simulink model "extra_simulink_blocks"  (R2018a)
settings: Solver=VariableStepAuto  StartTime=0.0  StopTime=10.0  RelTol=1e-3
values from neighbouring files (symbols this model uses):
  a1 = 16.235    [QuadrotorConstants.m]    (also in QuadrotorConstants.mat; TuningParameters.mat)
  a2 = 17.912    [QuadrotorConstants.m]    (also in QuadrotorConstants.mat; TuningParameters.mat)
  a3 = 17.914    [QuadrotorConstants.m]    (also in QuadrotorConstants.mat; TuningParameters.mat)
  a4 = 18.161    [QuadrotorConstants.m]    (also in QuadrotorConstants.mat; TuningParameters.mat)
  b1 = -0.5036    [QuadrotorConstants.m]    (also in QuadrotorConstants.mat; TuningParameters.mat)
  b2 = -12.728    [QuadrotorConstants.m]    (also in QuadrotorConstants.mat; TuningParameters.mat)
  b3 = -6.5646    [QuadrotorConstants.m]    (also in QuadrotorConstants.mat; TuningParameters.mat)
  b4 = -7.4637    [QuadrotorConstants.m]    (also in QuadrotorConstants.mat; TuningParameters.mat)
  bb = 2.6846e-07    [QuadrotorConstants.m]    (also in QuadrotorConstants.mat; TuningParameters.mat)
  c = 0.0002    [QuadrotorConstants.m]    (also in QuadrotorConstants.mat; TuningParameters.mat)
  c_mi_x = 1.70    (= 1.7)    [QuadrotorConstants.m]    (also in QuadrotorConstants.mat; TuningParameters.mat)
  c_mi_y = 1.70    (= 1.7)    [QuadrotorConstants.m]    (also in QuadrotorConstants.mat; TuningParameters.mat)
  c_mi_z = 0.40    (= 0.4)    [QuadrotorConstants.m]    (also in QuadrotorConstants.mat; TuningParameters.mat)
  co_x = 1.7    [QuadrotorConstants.m]    (also in QuadrotorConstants.mat; TuningParameters.mat)
  co_y = 1.7    [QuadrotorConstants.m]    (also in QuadrotorConstants.mat; TuningParameters.mat)
  co_z = 3    [QuadrotorConstants.m]    (also in QuadrotorConstants.mat; TuningParameters.mat)
  d = 0.0071    [QuadrotorConstants.m]    (also in QuadrotorConstants.mat; TuningParameters.mat)
  d_omega_R10 = V1_WP    [InitialConditions.m]    (also in TuningParameters.mat = 0.286149195881)
  d_omega_R20 = V2_WP    [InitialConditions.m]    (also in TuningParameters.mat = 0.941828505757)
  d_omega_R30 = V3_WP    [InitialConditions.m]    (also in TuningParameters.mat = 0.597668426656)
  d_omega_R40 = V4_WP    [InitialConditions.m]    (also in TuningParameters.mat = 0.639046979523)
  dd = 2.4481e-03    (= 0.0024481)    [QuadrotorConstants.m]    (also in QuadrotorConstants.mat; TuningParameters.mat)
  dfi_0 = 0    [InitialConditions.m]    (also in TuningParameters.mat)
  disturbancey = 0    [runMain.m]
  disturbancez = 0    [runMain.m]
  dpsi_0 = 0    [InitialConditions.m]    (also in TuningParameters.mat)
  dtheta_0 = 0    [InitialConditions.m]    (also in TuningParameters.mat)
  dx_0 = 0    [InitialConditions.m]    (also in TuningParameters.mat)
  dy_0 = 0    [InitialConditions.m]    (also in TuningParameters.mat)
  dz_0 = 5    [InitialConditions.m]    (also in TuningParameters.mat)
  f = 5e-6    (= 5e-06)    [QuadrotorConstants.m]    (also in QuadrotorConstants.mat; TuningParameters.mat; animateQuadrotor.m = getframe; animateQuadrotorConstant.m = getframe)
  fi_0 = pi    (= 3.14159265359)    [InitialConditions.m]    (also in TuningParameters.mat)
  g = 0.0008    [QuadrotorConstants.m]    (also in QuadrotorConstants.mat; TuningParameters.mat)
  ga = 9.807    [QuadrotorConstants.m]    (also in QuadrotorConstants.mat; TuningParameters.mat)
  h = -0.0282    [QuadrotorConstants.m]    (also in QuadrotorConstants.mat; TuningParameters.mat)
  Ixx = 2.1385*1    (= 2.1385)    [QuadrotorConstants.m]    (also in QuadrotorConstants.mat; TuningParameters.mat)
  Iyy = Ixx    (= 2.1385)    [QuadrotorConstants.m]    (also in QuadrotorConstants.mat; TuningParameters.mat)
  Izz = 3.7479*1    (= 3.7479)    [QuadrotorConstants.m]    (also in QuadrotorConstants.mat; TuningParameters.mat)
  Jr = 4.86851*0.1    (= 0.486851)    [QuadrotorConstants.m]    (also in QuadrotorConstants.mat; TuningParameters.mat)
  L = 0.422    [QuadrotorConstants.m]    (also in QuadrotorConstants.mat; TuningParameters.mat)
  m = 2.1    [QuadrotorConstants.m]    (also in QuadrotorConstants.mat; TuningParameters.mat)
  psi_0 = 0    [InitialConditions.m]    (also in TuningParameters.mat)
  Tau = 0.1    [QuadrotorConstants.m]    (also in QuadrotorConstants.mat; TuningParameters.mat)
  theta_0 = 0    [InitialConditions.m]    (also in TuningParameters.mat)
  x_0 = 0    [InitialConditions.m]    (also in TuningParameters.mat)
  XDes = [t,xdes,dxdes,ydes,dydes,zdes,dzdes,phides,dphides,thetades,dthetades,psides,dpsides]    [runMain.m]
  y_0 = 0    [InitialConditions.m]    (also in TuningParameters.mat)
  z_0 = 10    [InitialConditions.m]    (also in TuningParameters.mat)
undefined symbols (not defined in the file or in its folder): maxdz, sigbuilder_block, X, Y, Z
libraries: sm_lib x34, nesl_utility x21
(part 2 of 2)

== system extra_simulink_blocks/Dynamics1/Body dynamics ==
  U1 : Inport
  U2 : Inport  Port=2
  U3 : Inport  Port=3
  U4 : Inport  Port=4
  Omega : Inport  Port=5
  Mux : Mux  Inputs=6
  Pitch Stability : Subsystem
  Position Stability : Subsystem
  Roll Stability : Subsystem
  Yaw Stability : Subsystem
  Position : Outport
  Orientation : Outport  Port=2
  wires:
  U4/1 -> Yaw Stability/1(U4)
  U3/1 -> Pitch Stability/3(U3)
  U1/1 -> Position Stability/1(U1)
  U2/1 -> Roll Stability/2(U2)
  Omega/1 -> Pitch Stability/2(SumYRtrSpd), Roll Stability/1(SumXRtrSpd)
  Roll Stability/1(Phi) -> Mux/1, Position Stability/2(fi)
  Pitch Stability/1(Theta) -> Position Stability/3(theta), Mux/3
  Yaw Stability/1(Psi) -> Position Stability/4(psi), Mux/5
  Roll Stability/2(dPhi) -> Mux/2, Yaw Stability/2(dPhi), Pitch Stability/1(dPhi)
  Yaw Stability/2(dPsi) -> Roll Stability/4(dPsi), Pitch Stability/4(dPsi), Mux/6
  Pitch Stability/2(dTheta) -> Yaw Stability/3(dTheta), Roll Stability/3(dTheta), Mux/4
  Position Stability/1(Position) -> Position/1
  Mux/1 -> Orientation/1

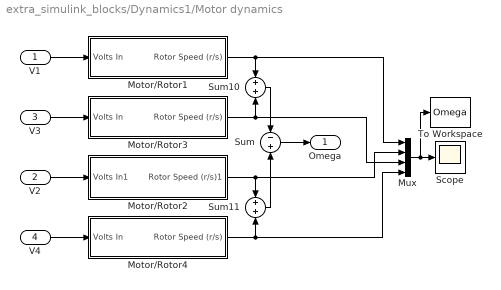
== system extra_simulink_blocks/Dynamics1/Motor dynamics ==
  V1 : Inport
  V2 : Inport  Port=2
  V3 : Inport  Port=3
  V4 : Inport  Port=4
  Motor/Rotor1 : Subsystem
  Motor/Rotor2 : Subsystem
  Motor/Rotor3 : Subsystem
  Motor/Rotor4 : Subsystem
  Mux : Mux
  Scope : Scope
  Sum : Sum  Inputs=-+
  Sum10 : Sum  Inputs=+|+
  Sum11 : Sum  Inputs=+|+
  To Workspace : ToWorkspace  VariableName=Omega  SaveFormat=Timeseries  SampleTime=-1
  Omega : Outport
  wires:
  Sum11/1 -> Sum/2
  Sum10/1 -> Sum/1
  Motor/Rotor4/1(Rotor Speed (r/s)) -> Mux/4, Sum11/2
  Motor/Rotor3/1(Rotor Speed (r/s)) -> Mux/3, Sum10/2
  Motor/Rotor2/1(Rotor Speed (r/s)1) -> Mux/2, Sum11/1
  Motor/Rotor1/1(Rotor Speed (r/s)) -> Mux/1, Sum10/1
  Sum/1 -> Omega/1
  V1/1 -> Motor/Rotor1/1(Volts In)
  V4/1 -> Motor/Rotor4/1(Volts In)
  V3/1 -> Motor/Rotor3/1(Volts In)
  V2/1 -> Motor/Rotor2/1(Volts In1)
  Mux/1 -> To Workspace/1, Scope/1

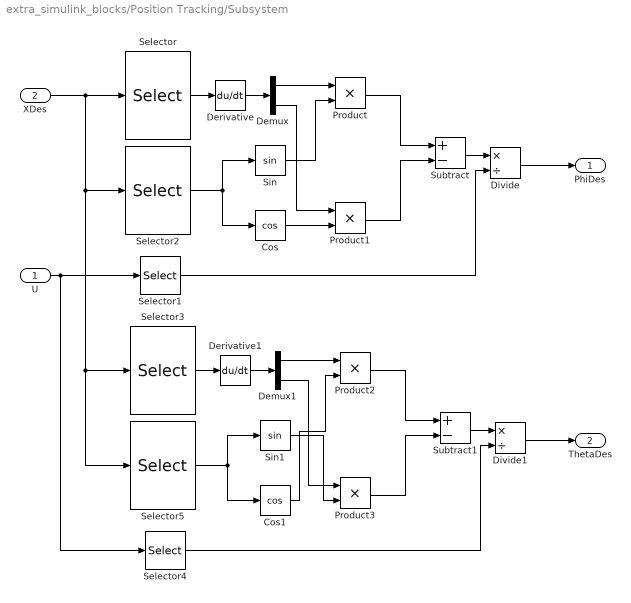
== system extra_simulink_blocks/Position Tracking/Subsystem ==
  U : Inport
  XDes : Inport  Port=2
  Cos : Trigonometry  Operator=cos
  Cos1 : Trigonometry  Operator=cos
  Demux : Demux  Outputs=2
  Demux1 : Demux  Outputs=2
  Derivative : Derivative
  Derivative1 : Derivative
  Divide : Product  Inputs=*/
  Divide1 : Product  Inputs=*/
  Product{,1..3} (4 alike) : Product
  Selector : Selector  InputPortWidth=12  IndexOptions=Index vector (dialog)  Indices=[2 4]  OutputSizes=1
  Selector1 : Selector  InputPortWidth=4  IndexOptions=Index vector (dialog)  Indices=[1]  OutputSizes=1
  Selector2 : Selector  InputPortWidth=12  IndexOptions=Index vector (dialog)  Indices=[11]  OutputSizes=1
  Selector3 : Selector  InputPortWidth=12  IndexOptions=Index vector (dialog)  Indices=[2 4]  OutputSizes=1
  Selector4 : Selector  InputPortWidth=4  IndexOptions=Index vector (dialog)  Indices=[1]  OutputSizes=1
  Selector5 : Selector  InputPortWidth=12  IndexOptions=Index vector (dialog)  Indices=[11]  OutputSizes=1
  Sin : Trigonometry
  Sin1 : Trigonometry
  Subtract : Sum  Inputs=+-
  Subtract1 : Sum  Inputs=+-
  PhiDes : Outport
  ThetaDes : Outport  Port=2
  wires:
  Derivative/1 -> Demux/1
  Selector/1 -> Derivative/1
  Demux/1 -> Product/1
  XDes/1 -> Selector5/1, Selector3/1, Selector2/1, Selector/1
  Cos/1 -> Product1/2
  Product/1 -> Subtract/1
  Product1/1 -> Subtract/2
  Subtract/1 -> Divide/1
  Divide/1 -> PhiDes/1
  Selector1/1 -> Divide/2
  Selector2/1 -> Cos/1, Sin/1
  Demux/2 -> Product1/1
  Sin/1 -> Product/2
  Selector3/1 -> Derivative1/1
  Product3/1 -> Subtract1/2
  Selector4/1 -> Divide1/2
  Product2/1 -> Subtract1/1
  U/1 -> Selector4/1, Selector1/1
  Divide1/1 -> ThetaDes/1
  Derivative1/1 -> Demux1/1
  Selector5/1 -> Cos1/1, Sin1/1
  Subtract1/1 -> Divide1/1
  Sin1/1 -> Product3/2
  Cos1/1 -> Product2/2
  Demux1/1 -> Product2/1
  Demux1/2 -> Product3/1

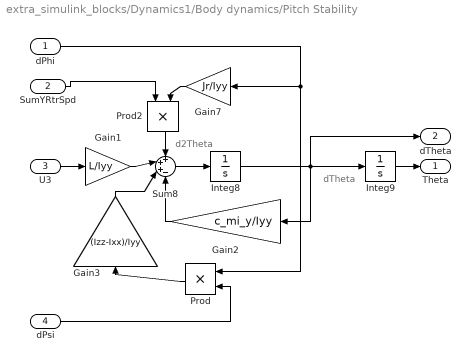
== system extra_simulink_blocks/Dynamics1/Body dynamics/Pitch Stability ==
  note: d2Theta
  note: dTheta
  dPhi : Inport
  SumYRtrSpd : Inport  Port=2
  U3 : Inport  Port=3
  dPsi : Inport  Port=4
  Gain1 : Gain  Gain=L/Iyy
  Gain2 : Gain  Gain=c_mi_y/Iyy
  Gain3 : Gain  Gain=(Izz-Ixx)/Iyy
  Gain7 : Gain  Gain=Jr/Iyy
  Integ8 : Integrator  InitialCondition=dtheta_0
  Integ9 : Integrator  InitialCondition=theta_0  UpperSaturationLimit=pi/2  LowerSaturationLimit=-pi/2
  Prod : Product  RndMeth=Zero
  Prod2 : Product  RndMeth=Zero
  Sum8 : Sum  Inputs=+++-
  Theta : Outport
  dTheta : Outport  Port=2
  wires:
  Gain2/1 -> Sum8/4
  dPhi/1 -> Prod/1, Gain7/1
  Integ9/1 -> Theta/1
  U3/1 -> Gain1/1
  SumYRtrSpd/1 -> Prod2/1
  dPsi/1 -> Prod/2
  Integ8/1 -> dTheta/1, Integ9/1, Gain2/1
  Sum8/1 -> Integ8/1
  Gain1/1 -> Sum8/2
  Gain7/1 -> Prod2/2
  Gain3/1 -> Sum8/3
  Prod/1 -> Gain3/1
  Prod2/1 -> Sum8/1

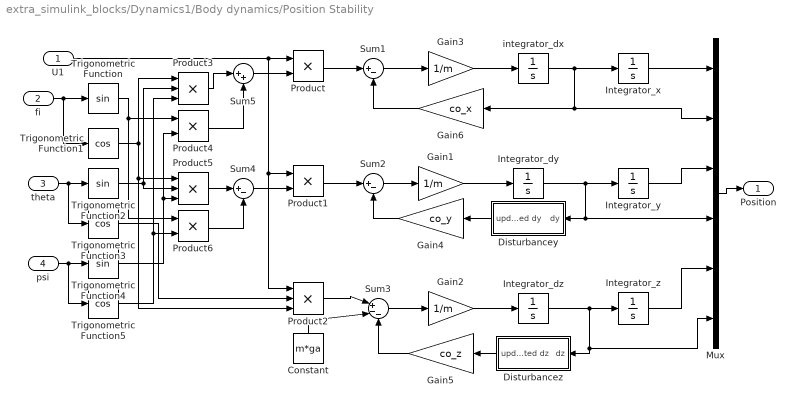
== system extra_simulink_blocks/Dynamics1/Body dynamics/Position Stability ==
  U1 : Inport
  fi : Inport  Port=2
  theta : Inport  Port=3
  psi : Inport  Port=4
  Constant : Constant  Value=m*ga
  Disturbancey : Subsystem
  Disturbancez : Subsystem
  Gain1 : Gain  Gain=1/m
  Gain2 : Gain  Gain=1/m
  Gain3 : Gain  Gain=1/m
  Gain4 : Gain  Gain=co_y
  Gain5 : Gain  Gain=co_z
  Gain6 : Gain  Gain=co_x
  Integrator_dy : Integrator  InitialCondition=dy_0  LimitOutput=on  UpperSaturationLimit=1000  LowerSaturationLimit=-1000
  Integrator_dz : Integrator  InitialCondition=dz_0  LimitOutput=on  UpperSaturationLimit=1000  LowerSaturationLimit=-1000
  Integrator_x : Integrator  InitialCondition=x_0
  Integrator_y : Integrator  InitialCondition=y_0
  Integrator_z : Integrator  InitialCondition=z_0
  Mux : Mux  Inputs=6
  Product{,1,4,6} (4 alike) : Product  RndMeth=Zero
  Product2 : Product  Inputs=3  RndMeth=Zero
  Product3 : Product  Inputs=3  RndMeth=Zero
  Product5 : Product  Inputs=3  RndMeth=Zero
  Sum1 : Sum  Inputs=|+-
  Sum2 : Sum  Inputs=|+-
  Sum3 : Sum  Inputs=|+--
  Sum4 : Sum  Inputs=|+-
  Sum5 : Sum  Inputs=|++
  Trigonometric Function : Trigonometry
  Trigonometric Function1 : Trigonometry  Operator=cos
  Trigonometric Function2 : Trigonometry
  Trigonometric Function3 : Trigonometry  Operator=cos
  Trigonometric Function4 : Trigonometry
  Trigonometric Function5 : Trigonometry  Operator=cos
  integrator_dx : Integrator  InitialCondition=dx_0  LimitOutput=on  UpperSaturationLimit=1000  LowerSaturationLimit=-1000
  Position : Outport
  wires:
  Gain5/1 -> Sum3/3
  Constant/1 -> Sum3/2
  Gain4/1 -> Sum2/2
  Sum3/1 -> Gain2/1
  Gain6/1 -> Sum1/2
  Product2/1 -> Sum3/1
  Sum2/1 -> Gain1/1
  Product1/1 -> Sum2/1
  Gain2/1 -> Integrator_dz/1
  Sum1/1 -> Gain3/1
  Product/1 -> Sum1/1
  U1/1 -> Product/1, Product1/1, Product2/1
  Integrator_x/1 -> Mux/1
  integrator_dx/1 -> Integrator_x/1, Mux/2, Gain6/1
  Integrator_dy/1 -> Integrator_y/1, Disturbancey/1(dy), Mux/4
  Integrator_dz/1 -> Integrator_z/1, Disturbancez/1(dz), Mux/6
  Gain1/1 -> Integrator_dy/1
  Gain3/1 -> integrator_dx/1
  Sum4/1 -> Product1/2
  Sum5/1 -> Product/2
  Product3/1 -> Sum5/1
  Product4/1 -> Sum5/2
  Product5/1 -> Sum4/1
  Product6/1 -> Sum4/2
  psi/1 -> Trigonometric Function4/1, Trigonometric Function5/1
  theta/1 -> Trigonometric Function2/1, Trigonometric Function3/1
  fi/1 -> Trigonometric Function/1, Trigonometric Function1/1
  Trigonometric Function/1 -> Product4/1, Product6/1
  Trigonometric Function1/1 -> Product3/1, Product5/1, Product2/3
  Trigonometric Function2/1 -> Product3/2, Product5/2
  Trigonometric Function5/1 -> Product3/3, Product6/2
  Trigonometric Function4/1 -> Product4/2, Product5/3
  Trigonometric Function3/1 -> Product2/2
  Integrator_y/1 -> Mux/3
  Integrator_z/1 -> Mux/5
  Mux/1 -> Position/1
  Disturbancez/1(updated dz) -> Gain5/1
  Disturbancey/1(updated dy) -> Gain4/1

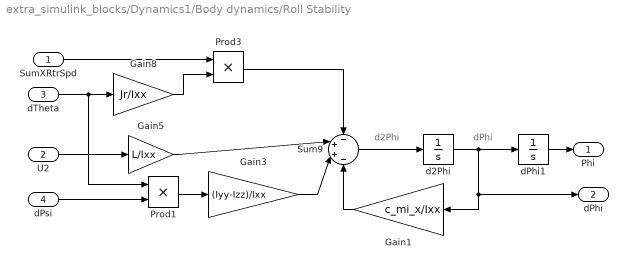
== system extra_simulink_blocks/Dynamics1/Body dynamics/Roll Stability ==
  note: d2Phi
  note: dPhi
  SumXRtrSpd : Inport
  U2 : Inport  Port=2
  dTheta : Inport  Port=3
  dPsi : Inport  Port=4
  Gain1 : Gain  Gain=c_mi_x/Ixx
  Gain3 : Gain  Gain=(Iyy-Izz)/Ixx
  Gain5 : Gain  Gain=L/Ixx
  Gain8 : Gain  Gain=Jr/Ixx
  Prod1 : Product  RndMeth=Zero
  Prod3 : Product  RndMeth=Zero
  Sum9 : Sum  Inputs=-++-
  d2Phi : Integrator  InitialCondition=dfi_0
  dPhi1 : Integrator  InitialCondition=fi_0  UpperSaturationLimit=pi/2  LowerSaturationLimit=-pi/2
  Phi : Outport
  dPhi : Outport  Port=2
  wires:
  dPsi/1 -> Prod1/2
  dTheta/1 -> Prod1/1, Gain8/1
  Prod3/1 -> Sum9/1
  SumXRtrSpd/1 -> Prod3/1
  Gain8/1 -> Prod3/2
  dPhi1/1 -> Phi/1
  U2/1 -> Gain5/1
  d2Phi/1 -> Gain1/1, dPhi/1, dPhi1/1
  Sum9/1 -> d2Phi/1
  Gain5/1 -> Sum9/2
  Gain1/1 -> Sum9/4
  Gain3/1 -> Sum9/3
  Prod1/1 -> Gain3/1

== system extra_simulink_blocks/Dynamics1/Body dynamics/Yaw Stability ==
  note: dPsi
  note: d2Psi
  U4 : Inport
  dPhi : Inport  Port=2
  dTheta : Inport  Port=3
  Gain : Gain  Gain=1/Izz
  Gain1 : Gain  Gain=c_mi_z
  Gain2 : Gain  Gain=Ixx-Iyy
  Integ10 : Integrator  InitialCondition=dpsi_0
  Integ11 : Integrator  InitialCondition=psi_0
  Product : Product  RndMeth=Zero
  Sum : Sum  Inputs=|++-
  Psi : Outport
  dPsi : Outport  Port=2
  wires:
  Sum/1 -> Gain/1
  U4/1 -> Sum/1
  Integ11/1 -> Psi/1
  Gain/1 -> Integ10/1
  Integ10/1 -> Gain1/1, dPsi/1, Integ11/1
  Gain1/1 -> Sum/3
  Gain2/1 -> Sum/2
  dPhi/1 -> Product/1
  dTheta/1 -> Product/2
  Product/1 -> Gain2/1

== system extra_simulink_blocks/Dynamics1/Motor dynamics/Motor//Rotor1 ==
  note: Omega1
      | (r/s)
  Volts In : Inport
  DragFcn1 : Fcn  Commented=on  Expr=dd*u^2
  Gain : Gain  Gain=1/Tau
  Integrator : Integrator  InitialCondition=d_omega_R10
  RtrSpdFcn1 : Fcn  Expr=a1*u+b1
  Saturation3 : Saturate  Commented=on  UpperLimit=1000  LowerLimit=-1000
  Saturation4 : Saturate  UpperLimit=250  LowerLimit=0
  Saturation8 : Saturate  Commented=on  UpperLimit=1000  LowerLimit=-1000
  Sum : Sum  Inputs=|+-
  ThrustFcn1 : Fcn  Commented=on  Expr=bb*u^2
  r/s 2 rpm : Gain  Commented=on  Gain=60/2/pi
  r/s 2 rpm1 : Gain  Commented=on  Gain=60/2/pi
  Rotor Speed (r/s) : Outport
  wires:
  Volts In/1 -> Sum/1
  Sum/1 -> Gain/1
  Integrator/1 -> RtrSpdFcn1/1, Sum/2
  Gain/1 -> Integrator/1
  DragFcn1/1 -> Saturation8/1
  RtrSpdFcn1/1 -> Saturation4/1
  ThrustFcn1/1 -> Saturation3/1
  Saturation4/1 -> Rotor Speed (r/s)/1, r/s 2 rpm1/1, r/s 2 rpm/1
  r/s 2 rpm/1 -> ThrustFcn1/1
  r/s 2 rpm1/1 -> DragFcn1/1

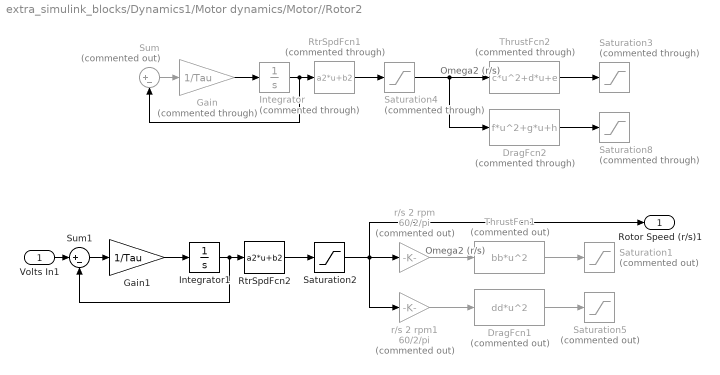
== system extra_simulink_blocks/Dynamics1/Motor dynamics/Motor//Rotor2 ==
  note: Omega2
      | (r/s)
  note: Omega2
      | (r/s)
  Volts In1 : Inport
  DragFcn1 : Fcn  Commented=on  Expr=dd*u^2
  DragFcn2 : Fcn  Commented=through  Expr=f*u^2+g*u+h
  Gain : Gain  Commented=through  Gain=1/Tau
  Gain1 : Gain  Gain=1/Tau
  Integrator : Integrator  Commented=through  InitialCondition=d_omega_R20
  Integrator1 : Integrator  InitialCondition=d_omega_R20
  RtrSpdFcn1 : Fcn  Commented=through  Expr=a2*u+b2
  RtrSpdFcn2 : Fcn  Expr=a2*u+b2
  Saturation1 : Saturate  Commented=on  UpperLimit=1000  LowerLimit=-1000
  Saturation2 : Saturate  UpperLimit=250  LowerLimit=0
  Saturation3 : Saturate  Commented=through  UpperLimit=1000  LowerLimit=-1000
  Saturation4 : Saturate  Commented=through  UpperLimit=1000  LowerLimit=-1000
  Saturation5 : Saturate  Commented=on  UpperLimit=1000  LowerLimit=-1000
  Saturation8 : Saturate  Commented=through  UpperLimit=1000  LowerLimit=-1000
  Sum : Sum  Commented=on  Inputs=|+-
  Sum1 : Sum  Inputs=|+-
  ThrustFcn1 : Fcn  Commented=on  Expr=bb*u^2
  ThrustFcn2 : Fcn  Commented=through  Expr=c*u^2+d*u+e
  r/s 2 rpm : Gain  Commented=on  Gain=60/2/pi
  r/s 2 rpm1 : Gain  Commented=on  Gain=60/2/pi
  Rotor Speed (r/s)1 : Outport
  wires:
  Sum/1 -> Gain/1
  Integrator/1 -> RtrSpdFcn1/1, Sum/2
  Gain/1 -> Integrator/1
  RtrSpdFcn1/1 -> Saturation4/1
  ThrustFcn2/1 -> Saturation3/1
  Saturation4/1 -> DragFcn2/1, ThrustFcn2/1
  DragFcn2/1 -> Saturation8/1
  DragFcn1/1 -> Saturation5/1
  Integrator1/1 -> RtrSpdFcn2/1, Sum1/2
  Gain1/1 -> Integrator1/1
  RtrSpdFcn2/1 -> Saturation2/1
  ThrustFcn1/1 -> Saturation1/1
  Volts In1/1 -> Sum1/1
  Sum1/1 -> Gain1/1
  Saturation2/1 -> Rotor Speed (r/s)1/1, r/s 2 rpm1/1, r/s 2 rpm/1
  r/s 2 rpm1/1 -> DragFcn1/1
  r/s 2 rpm/1 -> ThrustFcn1/1

== system extra_simulink_blocks/Dynamics1/Motor dynamics/Motor//Rotor3 ==
  note: Omega3
      | (r/s)
  Volts In : Inport
  DragFcn3 : Fcn  Commented=on  Expr=dd*u^2
  Gain : Gain  Gain=1/Tau
  Integrator : Integrator  InitialCondition=d_omega_R30
  RtrSpdFcn3 : Fcn  Expr=a3*u+b3
  Saturation3 : Saturate  Commented=on  UpperLimit=1000  LowerLimit=-1000
  Saturation4 : Saturate  UpperLimit=250  LowerLimit=0
  Saturation8 : Saturate  Commented=on  UpperLimit=1000  LowerLimit=-1000
  Sum : Sum  Inputs=|+-
  ThrustFcn3 : Fcn  Commented=on  Expr=bb*u^2
  r/s 2 rpm : Gain  Commented=on  Gain=60/2/pi
  r/s 2 rpm1 : Gain  Commented=on  Gain=60/2/pi
  Rotor Speed (r/s) : Outport
  wires:
  Volts In/1 -> Sum/1
  Sum/1 -> Gain/1
  Integrator/1 -> RtrSpdFcn3/1, Sum/2
  Gain/1 -> Integrator/1
  RtrSpdFcn3/1 -> Saturation4/1
  ThrustFcn3/1 -> Saturation3/1
  DragFcn3/1 -> Saturation8/1
  Saturation4/1 -> Rotor Speed (r/s)/1, r/s 2 rpm1/1, r/s 2 rpm/1
  r/s 2 rpm/1 -> ThrustFcn3/1
  r/s 2 rpm1/1 -> DragFcn3/1

== system extra_simulink_blocks/Dynamics1/Motor dynamics/Motor//Rotor4 ==
  note: Omega1
      | (r/s)
  Volts In : Inport
  DragFcn4 : Fcn  Commented=on  Expr=dd*u^2
  Gain : Gain  Gain=1/Tau
  Integrator : Integrator  InitialCondition=d_omega_R40
  RtrSpdFcn4 : Fcn  Expr=a4*u+b4
  Saturation3 : Saturate  Commented=on  UpperLimit=1000  LowerLimit=-1000
  Saturation4 : Saturate  UpperLimit=250  LowerLimit=0
  Saturation8 : Saturate  Commented=on  UpperLimit=1000  LowerLimit=-1000
  Sum : Sum  Inputs=|+-
  ThrustFcn4 : Fcn  Commented=on  Expr=bb*u^2
  r/s 2 rpm : Gain  Commented=on  Gain=60/2/pi
  r/s 2 rpm1 : Gain  Commented=on  Gain=60/2/pi
  Rotor Speed (r/s) : Outport
  wires:
  Volts In/1 -> Sum/1
  Sum/1 -> Gain/1
  Integrator/1 -> RtrSpdFcn4/1, Sum/2
  Gain/1 -> Integrator/1
  RtrSpdFcn4/1 -> Saturation4/1
  ThrustFcn4/1 -> Saturation3/1
  DragFcn4/1 -> Saturation8/1
  Saturation4/1 -> Rotor Speed (r/s)/1, r/s 2 rpm1/1, r/s 2 rpm/1
  r/s 2 rpm/1 -> ThrustFcn4/1
  r/s 2 rpm1/1 -> DragFcn4/1

== system extra_simulink_blocks/Dynamics1/Body dynamics/Position Stability/Disturbancey ==
  dy : Inport
  Constant1 : Constant  Value=disturbancey
  If : If  IfExpression=u1 == 1
  If Action Subsystem : Subsystem  TreatAsAtomicUnit=on
  If Action Subsystem1 : Subsystem  TreatAsAtomicUnit=on
  Merge : Merge
  updated dy : Outport
  wires:
  If Action Subsystem/1(updated dy) -> Merge/1
  If Action Subsystem1/1(updated dz) -> Merge/2
  Merge/1 -> updated dy/1
  If/2 -> If Action Subsystem1/Action
  Constant1/1 -> If/1
  If/1 -> If Action Subsystem/Action
  dy/1 -> If Action Subsystem/1(dy), If Action Subsystem1/1(dz)

== system extra_simulink_blocks/Dynamics1/Body dynamics/Position Stability/Disturbancez ==
  dz : Inport
  Constant1 : Constant  Value=disturbancez
  If : If  IfExpression=u1 == 1
  If Action Subsystem : Subsystem  TreatAsAtomicUnit=on
  If Action Subsystem1 : Subsystem  TreatAsAtomicUnit=on
  Merge : Merge
  updated dz : Outport
  wires:
  If Action Subsystem/1(updated dz) -> Merge/1
  If Action Subsystem1/1(updated dz) -> Merge/2
  Merge/1 -> updated dz/1
  If/2 -> If Action Subsystem1/Action
  Constant1/1 -> If/1
  If/1 -> If Action Subsystem/Action
  dz/1 -> If Action Subsystem/1(dz), If Action Subsystem1/1(dz)

== system extra_simulink_blocks/Dynamics1/Body dynamics/Position Stability/Disturbancey/If Action Subsystem ==
  dy : Inport
  Action Port : ActionPort
  add disturbance : Subsystem
  updated dy : Outport
  wires:
  dy/1 -> add disturbance/1(dy)
  add disturbance/1(updated dy) -> updated dy/1

== system extra_simulink_blocks/Dynamics1/Body dynamics/Position Stability/Disturbancey/If Action Subsystem1 ==
  dz : Inport
  Action Port : ActionPort
  updated dz : Outport
  wires:
  dz/1 -> updated dz/1

== system extra_simulink_blocks/Dynamics1/Body dynamics/Position Stability/Disturbancez/If Action Subsystem ==
  dz : Inport
  Action Port : ActionPort
  add disturbance : Subsystem
  updated dz : Outport
  wires:
  dz/1 -> add disturbance/1(dz)
  add disturbance/1(updated dz) -> updated dz/1

== system extra_simulink_blocks/Dynamics1/Body dynamics/Position Stability/Disturbancez/If Action Subsystem1 ==
  dz : Inport
  Action Port : ActionPort
  updated dz : Outport
  wires:
  dz/1 -> updated dz/1

== system extra_simulink_blocks/Dynamics1/Body dynamics/Position Stability/Disturbancey/If Action Subsystem/add disturbance ==
  dy : Inport
  Subtract : Sum  Inputs=-+
  "vwind " : Subsystem
  updated dy : Outport
  wires:
  dy/1 -> Subtract/2
  "vwind "/1(vwind) -> Subtract/1
  Subtract/1 -> updated dy/1

== system extra_simulink_blocks/Dynamics1/Body dynamics/Position Stability/Disturbancez/If Action Subsystem/add disturbance ==
  dz : Inport
  Subtract : Sum  Inputs=-+
  "vwind " : Subsystem
  updated dz : Outport
  wires:
  dz/1 -> Subtract/2
  "vwind "/1(vwind) -> Subtract/1
  Subtract/1 -> updated dz/1

== system extra_simulink_blocks/Dynamics1/Body dynamics/Position Stability/Disturbancey/If Action Subsystem/add disturbance/vwind  ==
  Signal Builder : Subsystem  Tag=STV Subsys  LoadFcn=sigbuilder_block('load');  StartFcn=sigbuilder_block('start');  StopFcn=sigbuilder_block('stop');  ClipboardFcn=sigbuilder_block('clipboard');  mask(Sigbuilder block){tuvar=[0:10]}
      mask help: Simulink:masks:SigbuilderBlock_MD
      mask init:
      | if ~strcmp(get_param(bdroot(gcbh),'SimulationStatus'),'stopped') tuvar = sigbuilder_block('maskInit'); end
      settings: CopyFcn=sigbuilder_block('copy');  DeleteFcn=sigbuilder_block('delete');  ModelCloseFcn=sigbuilder_block('modelClose');  PreSaveFcn=sigbuilder_block('preSave');  PauseFcn=sigbuilder_block('pause');  ContinueFcn=sigbuilder_block('continue');  NameChangeFcn=sigbuilder_block('namechange');  OpenFcn=sigbuilder_block('open',[394.2 102 550.8 400.2 ]);  CloseFcn=sigbuilder_block('close');
      mask Display: plot(0, 0, 100, 100,[2, 2, 32, 32, 2], [68, 8, 8, 68, 68],[32, 2], [38, 38], [32, 19, 2],[53, 60, 44], [32, 17, 17, 2],[16, 16, 31, 31]);txt = getActiveGroup(gcbh);text(2, 100, txt,'verticalAlignment', 'top');
  vwind : Outport
  wires:
  Signal Builder/1(Signal 1) -> vwind/1

== system extra_simulink_blocks/Dynamics1/Body dynamics/Position Stability/Disturbancez/If Action Subsystem/add disturbance/vwind  ==
  note: step down
  note: step up
  Add : Sum  Commented=on
  Signal Builder : Subsystem  Tag=STV Subsys  LoadFcn=sigbuilder_block('load');  StartFcn=sigbuilder_block('start');  StopFcn=sigbuilder_block('stop');  ClipboardFcn=sigbuilder_block('clipboard');  mask(Sigbuilder block){tuvar=[0:10]}
      mask help: Simulink:masks:SigbuilderBlock_MD
      mask init:
      | if ~strcmp(get_param(bdroot(gcbh),'SimulationStatus'),'stopped') tuvar = sigbuilder_block('maskInit'); end
      settings: CopyFcn=sigbuilder_block('copy');  DeleteFcn=sigbuilder_block('delete');  ModelCloseFcn=sigbuilder_block('modelClose');  PreSaveFcn=sigbuilder_block('preSave');  PauseFcn=sigbuilder_block('pause');  ContinueFcn=sigbuilder_block('continue');  NameChangeFcn=sigbuilder_block('namechange');  OpenFcn=sigbuilder_block('open',[437.6 199.2 550.4 400 ]);  CloseFcn=sigbuilder_block('close');
      mask Display: plot(0, 0, 100, 100,[2, 2, 32, 32, 2], [68, 8, 8, 68, 68],[32, 2], [38, 38], [32, 19, 2],[53, 60, 44], [32, 17, 17, 2],[16, 16, 31, 31]);txt = getActiveGroup(gcbh);text(2, 100, txt,'verticalAlignment', 'top');
  Step : Step  Commented=on  Time=2  After=maxdz  SampleTime=0
  Step1 : Step  Commented=on  Time=2.25  After=-maxdz  SampleTime=0
  vwind : Outport
  wires:
  Signal Builder/1(Signal 1) -> vwind/1
  Step/1 -> Add/1
  Step1/1 -> Add/2

== system extra_simulink_blocks/Dynamics1/Body dynamics/Position Stability/Disturbancey/If Action Subsystem/add disturbance/vwind /Signal Builder ==
  Demux : Demux  Tag=STV Demux  Outputs=1
  FromWs : FromWorkspace  Tag=STV FromWs  VariableName=tuvar  SampleTime=0
      SigBuilderData=|
      | common.afterFinalStr = 'Extrapolate'
      | common.sampleTime = 0
      | dataSet.timeRange = [0 10]
      | dataSet.name = 'Group 1'
      | sbobj.Groups.Name = 'Group 1'
      | sbobj.Groups.Signals.Name = 'Signal 1'
      | sbobj.Groups.Signals.XData = [0 2 2 2.001 10]
      | sbobj.Groups.Signals.YData = [0 0 10000 0 0]
  Signal 1 : Outport  Tag=STV Outport
  wires:
  Demux/1 -> Signal 1/1
  FromWs/1 -> Demux/1

== system extra_simulink_blocks/Dynamics1/Body dynamics/Position Stability/Disturbancez/If Action Subsystem/add disturbance/vwind /Signal Builder ==
  Demux : Demux  Tag=STV Demux  Outputs=1
  FromWs : FromWorkspace  Tag=STV FromWs  VariableName=tuvar  SampleTime=0
      SigBuilderData=|
      | common.afterFinalStr = 'Extrapolate'
      | common.sampleTime = 0
      | dataSet.timeRange = [0 10]
      | dataSet.name = 'Group 1'
      | sbobj.Groups.Name = 'Group 1'
      | sbobj.Groups.Signals.Name = 'Signal 1'
      | sbobj.Groups.Signals.XData = [0 2 2 2.001 10]
      | sbobj.Groups.Signals.YData = [0 0 10000 0 0]
  Signal 1 : Outport  Tag=STV Outport
  wires:
  Demux/1 -> Signal 1/1
  FromWs/1 -> Demux/1

== matlab function extra_simulink_blocks/Controller1/calculateU ==
  data: x input; u output; xd input; om input; s output
function [u,s] = fcn(x,xd,om)

% load parameters
p = load('QuadrotorConstants'); % Load quadrotor constants
t = load('TuningParameters');   % Load tuning parameters

% initialize memory for u and s
u = zeros(4,1);
s = zeros(4,1);

% store state into smaller variables
X   = [ x(5)  x(7)  x(9)   x(11)].';
dX  = [ x(6)  x(8)  x(10)  x(12)].';
Xd  = [xd(5) xd(7) xd(9)  xd(11)].';
% dXd = [xd(6) xd(8) xd(10) xd(12)].';

% find desired derivatives
dXd = (Xd-X)./t.tau;
% dXd(2:4) = 1e-6*dXd(2:4);
ddXd = (dXd-dX)./t.tau;

% sliding surfaces
s = t.lambda.*(Xd-X) + (dXd-dX);

% find the sign / sigmoid of sliding surfaces
sigma = tanh(s);

% find the derivatives of sliding surfaces
ds = - t.K.*sigma - t.eta.*s;

% find the EOMs from the sliding surfaces
% ddx = zeros(4,1);
ddX = - ds + t.lambda.*(dXd - dX) + ddXd;

% find which state should be controlled
% s(~cont) = 0;

% find the inputs
% if s(1) ~= 0
%     u(1) = ( p.m/cos(X(2))/cos(X(3)) ) * ...
%         ( p.ga + ddX(1));
% end
% if s(2) ~= 0
%     u(2) = (p.Ixx/p.L) * ( - ((p.Iyy-p.Izz)/(p.Ixx))*dX(3)*dX(4) + ...
%         (p.Jr/p.Ixx)*dX(3)*om + ddX(2) );
% end
% if s(3) ~= 0 
%     u(3) = (p.Iyy/p.L) * ( - ((p.Izz-p.Ixx)/(p.Iyy))*dX(2)*dX(4) - ...
%         (p.Jr/p.Ixx)*dX(2)*om + ddX(3) );
% end
% if s(4) ~= 0
%     u(4) = (p.Izz/p.L) * ( - ((p.Ixx-p.Iyy)/(p.Izz))*dX(2)*dX(3) + ddX(4));
% end


u(1) = ( p.m/cos(X(2))/cos(X(3)) ) * ( p.ga + ddX(1) );
u(2) = (p.Ixx/p.L) * ( - ((p.Iyy-p.Izz)/(p.Ixx))*dX(3)*dX(4) + (p.Jr/p.Ixx)*dX(3)*om + ddX(2) );
u(3) = (p.Iyy/p.L) * ( - ((p.Izz-p.Ixx)/(p.Iyy))*dX(2)*dX(4) - (p.Jr/p.Iyy)*dX(2)*om + ddX(3) );
u(4) = (p.Izz/p.L) * ( - ((p.Ixx-p.Iyy)/(p.Izz))*dX(2)*dX(3) + ddX(4));

end

== matlab function extra_simulink_blocks/Controller1/findVolts/MATLAB Function ==
  data: U input; Omegas output
function Omegas = fcn(U)

% initialize memory for omega
Omegas = zeros(4,1);

% coefficients
bb = 2.6846e-07;
dd = 2.4481e-08;

% linear system matrix
A = [bb bb bb bb; 0 -bb 0 bb; -bb 0 bb 0; -dd dd -dd dd];

% Omegas = A\U;
% 
% for i = 1:length(Omegas)
%     Omegas(i) = real(Omegas(i));
% end
% 
% Omegas = sqrt(Omegas);


% square root all of the omega values
Omegas = sqrt((A\U).*sign(A\U));
% if sum(imag(complex(A\U))) ~= 0
% Omegas = sqrt(complex(real(A\U),imag(A\U)));%.*sign(A\U));
% else
% Omegas = sqrt(A\U);%.*sign(A\U));
% end
end
